simulink library "tqd"  (R2021b)
settings: Solver=VariableStepAuto  StartTime=0.0  StopTime=10.0  RelTol=1e-3
undefined symbols (not defined in the file or in its folder): ATQD_AccelLimitInRange_X_rpm, ATQD_AccelLimitInRange_Y_Nm, ATQD_AccelLimitOvrKi_X_Nm, ATQD_AccelLimitOvrKp_X_Nm, ATQD_BOSMapD_X_rpm, ATQD_BOSMapD_Y_pct, ATQD_BOSMapR_X_rpm, ATQD_BOSMapR_Y_pct, ATQD_HVBCurrSmooth_X_A, ATQD_LHMTqMapDLC_X_rpm, ATQD_LHMTqMapDLC_Y_pct, ATQD_LHMTqMapRLC_X_rpm, ATQD_LHMTqMapRLC_Y_pct, ATQD_NormalMapDLC_X_rpm, ATQD_NormalMapDLC_Y_pct, ATQD_NormalTqDecSR_X_rpm, ATQD_NormalTqDecSR_Y_Nm, ATQD_NormalTqIncSR_X_rpm, ATQD_NormalTqIncSR_Y_Nm, ATQD_OPDMapRLC_X_rpm, ATQD_OPDMapRLC_Y_pct, ATQD_RollRegTorReq_X_rpm, ATQD_RollRegTorReq_Y_enum, ATQD_VehSpdLimitInRange_X_rpm, ATQD_VehSpdLimitInRange_Y_Nm, ATQD_VehSpdLimitOvrKi_X_Nm, ATQD_VehSpdLimitOvrKp_X_Nm, EIGHT_INT, ENUM_BRAKEPEDAL_PRESSED, ENUM_BRAKEPEDAL_RELEASED, ENUM_COMBOKEY_DOWN, ENUM_COMBOKEY_M1, ENUM_COMBOKEY_M2, ENUM_COMBOKEY_NONE, ENUM_COMBOKEY_RKNEE, ENUM_COMBOKEY_STOPLV, ENUM_COMBOKEY_UP, ENUM_CP2VKNEEREQ_REQUEST, ENUM_CP2VNLVREQ_LEVEL1, ENUM_CP2VNLVREQ_LEVEL2, ENUM_CP2VNLVREQ_LOWER, ENUM_CP2VNLVREQ_STOPLV, ENUM_CP2VNLVREQ_UPPER, ENUM_CREEPIND_DISABLE, ENUM_CREEPIND_READY, ENUM_CREEPIND_RUNNING, ENUM_CREEPIND_WARNING, ENUM_DRIVELINERELEASE_RELEASE, ENUM_EBSTORQUERWQ_LIMIT, ENUM_EBSTORQUERWQ_TORQUE, ENUM_ECPVCUDRM_CONFORT, ENUM_ECPVCUDRM_ECO, ENUM_ECPVCUDRM_NORMAL, ENUM_ECPVCUDRM_NOTAVAILABLE, ENUM_EMTqModeDrvBrk_Accel, ENUM_EMTqModeDrvBrk_Brake, ENUM_EMTqModeDrvBrk_Coast, ENUM_ETC2ACTDRIVEDIR_BACKWARD, ENUM_ETC2ACTDRIVEDIR_FORWARD, ENUM_ETC2ACTDRIVEDIR_STILL ... (+341)
libraries: simulink x109, hcu_lib x67
(part 3 of 13)

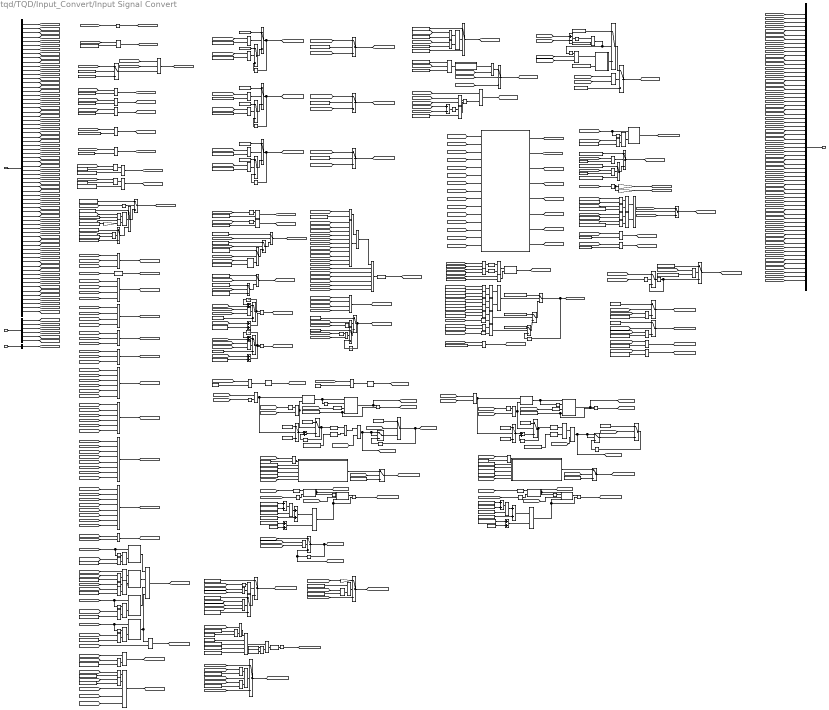
== system tqd/TQD/Input_Convert/Input Signal Convert ==
  note: VCU Vehicle Speed
  note: Motor Speed with Direction
  note: EBS Torque Control Determination
  note: Actual Driver Mode Determination
  note: Available Torque Calculation
  note: Target Shafter Speed Determination
  note: Gear Shifter Transfer Determination
  note: Gear Limitation with DMS Lost Communication
  note: DDM for DCQ
  note: Combo Key
  note: Engineering Mode Detection
  note: MCU Speed High Value Determination
  note: Actual Driving Direction Determination
  note: Power Limit/Gear Flash Indication Determination
  note: EBS Torque Request Determination
  note: IGN Active
  note: EV Drive Ready Judgment
  note: Gear Request Determination
  note: Door Open Judgment
  note: Brake Switch On
  note: Acceleration Pedal Depressed
  note: SCP Door Status
  note: Torque Source Determination
  BSCPIn_outputs : Inport
  BDCQ_Function_outputs : Inport  Port=2
  BDCQ_main_outputs : Inport  Port=3
  AND{,1..7,11..17} (15 alike) : Logic  AllPortsSameDT=off  OutDataTypeStr=boolean
  AND10 : Logic  Operator=OR  AllPortsSameDT=off  OutDataTypeStr=boolean
  AND18 : Logic  Inputs=3  AllPortsSameDT=off  OutDataTypeStr=boolean
  AND8 : Logic  Inputs=3  AllPortsSameDT=off  OutDataTypeStr=boolean
  AND9 : Logic  Operator=OR  AllPortsSameDT=off  OutDataTypeStr=boolean
  Abs{,1,5..6} (4 alike) : Abs
  Add{,1..3,7..14} (12 alike) : Sum
  Add5 : Sum  Inputs=+-
  Add6 : Sum  Inputs=+-
  "Big Mike Combo V2 " : Subsystem  TreatAsAtomicUnit=on
      settings: RTWSystemCode=Nonreusable function
  Bus Creator : BusCreator  Inputs=65
  Bus Selector : BusSelector  OutputSignals=task_time_s,VDHP_LowIdleAccPedal_flg,VINP_EBSBrakeSw_enum,VINP_TransReqGear_enum,VPMM_DrivelineRelease_enum,VPSA_Keystatus_enum,VINP_EM1ReqTorqLimDriv_pct,VINP_EM1ReqTorqLimBrk_pct,VPMM_SysPowerMode_enum,VDMM_DTCBMSRlyNoFB_flg,VDMM_DTCDCDCInverNoFB_flg,VDMM_DTCEACInverNoFB_flg,VDMM_DTCEACRlyNoFB_flg,VDMM_DTCEHPSInverNoFB_flg,VDMM_DTCEHPSRlyNoFB_flg,VDMM_DTCMCUHVRlyNoFB_flg,VDMM_DTCMCUIGBNoFB_flg,VDMM_DTCMCUCtrlMdNoFB_flg,VDMM_DTCACHVRlyNoFB_flg,VDMM_DTCMotorSpdNoFB_flg,VDMM_DTCMotorTrqNoFB_flg,VDMM_DTCDCDCRlyNoFB_flg,VDMM_DTCLostTC1_flg,VDMM_DTCDMSRCIncorrect_flg,VINP_MotorSpd_rpm,VINP_MotorSpdValid_flg,VINP_ECPVCUSpdLim_kph,VINP_ECPVCUSpdLimSw_flg,VINP_ParkBrakeSW_flg,VINP_BrakePedalPos_pct,VDHP_ActAPSPosn_pct,VDMM_DTCLostB2VST1_flg,VDMM_DTCLostB2VST2_flg,VDMM_DTCLostB2VCurrentLimit_flg,VDMM_DTCLostEMCEM1_flg,VDMM_DTCLostEBC1_flg,VDMM_DTCLostEBC2_flg,VDMM_DTCLostEBC5_flg,VDMM_ActLostEMCEM1_flg,VDMM_ActLostEBC1_flg,VDMM_ActLostEBC2_flg,VDMM_ActLostEBC5_flg,VDMM_ActLostMCUSta1_flg,VDMM_ActLostMCUSta2_flg,VDMM_ActLostMCUSta3_flg,VDMM_ActLostB2VST1_flg,VDMM_ActLostB2VST2_flg,VDMM_ActLostB2VCurrentLimit_flg,VDMM_DTCBCURCIncorrect_flg,VDMM_DTCPDURCIncorrect_flg,VINP_ECPVCUDRM_enum,VDMM_CAN1BUSOFF_flg,VINP_EM1OvrCtrlMDriv_enum,VINP_EM1OvrCtrlMBrk_enum,VDMM_EBSRCIncorrect_flg,VINP_FRHalbrakeReq_enum,VINP_MDHalbrakeReq_enum,VINP_TDHalbrakeReq_enum,VBCM_FDCBCMFDoorSta_flg,VBCM_FDCBCMMDoorSta_flg,VBCM_FDCBCMRDoorSta_flg,VACC_ASC2NLvReqFA_enum,VACC_ASC2NLvReqRA_enum,VACC_ASC2KneeReqRSide_flg,VACC_ASC2KneeReqFA_flg,VACC_ASC2KneeReqRA_flg,VBCM_FDCBCMFDCloseSVCmd_flg,VBCM_FDCBCMFDOpenSVCmd_flg,VINP_FASpeed_kph,VINP_CANMsgValidEBC2_flg
  Bus Selector1 : BusSelector  OutputSignals=VTQD_GearActualPosn_enum,VTQD_ParkingProtectWarning_flg,VTQD_TorqLimDoorOpn_flg,VTQD_VCUMCUCtrlMdTQD_enum,VTQD_TMTqCapMot_Nm,VTQD_TMTqCapGen_Nm
  Bus Selector2 : BusSelector  OutputSignals=VTQD_RrRampTq_Nm
  Constant{,2,71,73} (4 alike) : Constant  Value=ZERO_FLOAT
  Constant1 : Constant  Value=ENUM_GEARSHIFTPOSN_D
  Constant10 : Constant  Value=ENUM_BRAKEPEDAL_PRESSED
  Constant100 : Constant  Value=ENUM_MCUCTRLMODE_TORQUE
  Constant101 : Constant  Value=ENUM_GEARACTUALPOSN_R
  Constant102 : Constant  Value=KTQD_AbsoluteMotorSpdDir_flg
  Constant103 : Constant  Value=EPS
  Constant104 : Constant  Value=ENUM_GEARACTUALPOSN_N
  Constant105 : Constant  Value=ENUM_GEARACTUALPOSN_R
  Constant106 : Constant  Value=ENUM_GEARSHIFTPOSN_D
  Constant107 : Constant  Value=ENUM_GEARSHIFTPOSN_INVALID
  Constant108 : Constant  Value=ENUM_GEARSHIFTPOSN_N
  Constant109 : Constant  Value=ENUM_GEARSHIFTPOSN_R
  Constant11 : Constant  Value=ONE_PERCENT
  Constant110 : Constant  Value=KTQD_GearFlashSetTime_s
  Constant111 : Constant  Value=EPS
  Constant112 : Constant  Value=ENUM_GEARSHIFTPOSN_N
  Constant113 : Constant  Value=ENUM_GEARSHIFTPOSN_R
  Constant114 : Constant  Value=KTQD_VehSpdGearRatio_ratio
  Constant115 : Constant  Value=KTQD_ActDrvDirMotorSpdLimit_rpm  OutDataTypeStr=single
  Constant116 : Constant  Value=KTQD_GearFlashSetTime_s
  Constant117 : Constant  Value=EPS  OutDataTypeStr=single
  Constant118 : Constant  Value=KTQD_VehSpdTireFactor_Factor
  Constant119 : Constant  Value=KTQD_VehSpdTireDiameter_m
  Constant12 : Constant  Value=KTQD_MCUMaxRefTorq_Nm
  Constant120 : Constant  Value=KTQD_VehSpdADJFactor_Factor
  Constant{121,206,210,215,220} (5 alike) : Constant  Value=TRUE
  Constant122 : Constant  Value=SIXTY
  Constant123 : Constant  Value=THOUSAND
  Constant124 : Constant  Value=EPS  OutDataTypeStr=single
  Constant125 : Constant  Value=KTQD_TMSpd2FASpd_kph
  Constant126 : Constant  Value=KTQD_VCUVehSpdErr_kph
  Constant13 : Constant  Value=ENUM_GEARACTUALPOSN_D  OutDataTypeStr=Inherit: Inherit via back propagation
  Constant14 : Constant  Value=ENUM_GEARACTUALPOSN_P  OutDataTypeStr=Inherit: Inherit via back propagation
  Constant15 : Constant  Value=KTQD_EnLVChrgModekeyDet_s  OutDataTypeStr=single
  Constant16 : Constant  Value=ENUM_TARGETGEAR_DRIVE
  Constant17 : Constant  Value=ENUM_TARGETGEAR_NEUTRAL
  Constant176 : Constant  Value=uint8(6)
  Constant18 : Constant  Value=ENUM_TARGETGEAR_REVERSE
  Constant189 : Constant  Value=ENUM_VEHACTDRVDIR_ERROR
  Constant19 : Constant  Value=KTQD_EnLVChrgModeUION_s  VectorParams1D=off
  Constant198 : Constant  Value=KTQD_SpdLimSatHi_kph
  Constant20 : Constant  Value=KTQD_TDDoorSW_flg
  Constant200 : Constant  Value=KTQD_SpdLimSatLo_kph
  Constant202 : Constant  Value=KTQD_SpdLimDiv_rpm
  Constant{3,21,49..50,90,98,203,211,216,221} (10 alike) : Constant  Value=FALSE
  Constant204 : Constant  Value=KTQD_SpdLimDiv_rpm
  Constant205 : Constant  Value=KTQD_SpdLimIndFlash_cnt
  Constant207 : Constant  Value=KTQD_DoorStaSourceSW_flg
  Constant208 : Constant  Value=ENUM_HALBRAKEREQ_NOTACTIVE
  Constant209 : Constant  Value=ENUM_HALBRAKEREQ_ACTIVE
  Constant212 : Constant  Value=KTQD_DoorStaSourceSW_flg
  Constant213 : Constant  Value=ENUM_HALBRAKEREQ_NOTACTIVE
  Constant214 : Constant  Value=ENUM_HALBRAKEREQ_ACTIVE
  Constant217 : Constant  Value=KTQD_DoorStaSourceSW_flg
  Constant218 : Constant  Value=ENUM_HALBRAKEREQ_NOTACTIVE
  Constant219 : Constant  Value=ENUM_HALBRAKEREQ_ACTIVE
  Constant22 : Constant  Value=ENUM_KEYSTATUS_START
  Constant23 : Constant  Value=KTQD_DisLVChrgModeKeyDet_c  VectorParams1D=off
  Constant{24,44,52,55} (4 alike) : Constant  Value=ZERO_INT
  Constant242 : Constant  Value=ENUM_ECPVCUDRM_ECO
  Constant243 : Constant  Value=ENUM_ECPVCUDRM_CONFORT
  Constant244 : Constant  Value=KTQD_ECOComfortSpdLim_rpm
  Constant25 : Constant  Value=KTQD_EnLVChrgModeUIOFF_s  VectorParams1D=off
  Constant26 : Constant  Value=KTQD_EnLVChrgModeUIFlash_cnt  VectorParams1D=off
  Constant27 : Constant  Value=ENUM_DRIVELINERELEASE_RELEASE
  Constant28 : Constant  Value=KTQD_EnLVChrgModeUIWait_s  VectorParams1D=off
  Constant29 : Constant  Value=KTQD_EnLVChrgModeUION_s  VectorParams1D=off
  Constant30 : Constant  Value=KTQD_EnLVChrgModeUIOFF_s  VectorParams1D=off
  Constant31 : Constant  Value=KTQD_EnLVChrgModeUIFlash_cnt  VectorParams1D=off
  Constant32 : Constant  Value=KTQD_EnLVChrgModeUIWait_s  VectorParams1D=off
  Constant{33,47..48,54} (4 alike) : Constant  Value=ONE_INT
  Constant34 : Constant  Value=KTQD_EnLVChrgModeUITimes_cnt  VectorParams1D=off
  Constant35 : Constant  Value=FALSE  VectorParams1D=off
  Constant36 : Constant  Value=KTQD_DisLVChrgModeUION_s  VectorParams1D=off
  Constant37 : Constant  Value=KTQD_DisLVChrgModeUIOFF_s  VectorParams1D=off
  Constant38 : Constant  Value=KTQD_DisLVChrgModeUIFlash_cnt  VectorParams1D=off
  Constant39 : Constant  Value=KTQD_DisLVChrgModeUIWait_s  VectorParams1D=off
  Constant4 : Constant  Value=uint8(7)
  Constant40 : Constant  Value=KTQD_DisLVChrgModeUION_s  VectorParams1D=off
  Constant41 : Constant  Value=KTQD_DisLVChrgModeUIOFF_s  VectorParams1D=off
  Constant42 : Constant  Value=KTQD_DisLVChrgModeUIFlash_cnt  VectorParams1D=off
  Constant43 : Constant  Value=KTQD_DisLVChrgModeUIWait_s  VectorParams1D=off
  Constant45 : Constant  Value=KTQD_DisLVChrgModeUITimes_cnt  VectorParams1D=off
  Constant46 : Constant  Value=FALSE  VectorParams1D=off
  Constant5 : Constant  Value=KTQD_MCUMaxRefTorq_Nm
  Constant51 : Constant  Value=KTQD_EnLVChrgModeKeyDet_cnt
  Constant53 : Constant  Value=KTQD_DisLVChrgModeKeyDet_s  OutDataTypeStr=single
  Constant56 : Constant  Value=ENUM_GEARACTUALPOSN_R  OutDataTypeStr=Inherit: Inherit via back propagation
  Constant57 : Constant  Value=KTQD_VCUMCUDemHiPosVal_rpm
  Constant58 : Constant  Value=ENUM_TMROTATEDIRECTREQ_NONE  OutDataTypeStr=uint8
  Constant59 : Constant  Value=ENUM_TMROTATEDIRECTREQ_FWD  OutDataTypeStr=uint8
  Constant6 : Constant  Value=ONE_PERCENT
  Constant60 : Constant  Value=ENUM_TMROTATEDIRECTREQ_REV  OutDataTypeStr=uint8
  Constant61 : Constant  Value=KTQD_RotaDirRngUpTq_Nm
  Constant62 : Constant  Value=ENUM_GEARACTUALPOSN_R  OutDataTypeStr=Inherit: Inherit via back propagation
  Constant63 : Constant  Value=ENUM_GEARACTUALPOSN_D  OutDataTypeStr=Inherit: Inherit via back propagation
  Constant64 : Constant  Value=ENUM_TMROTATEDIRECTREQ_NONE  OutDataTypeStr=Inherit: Inherit via back propagation
  Constant65 : Constant  Value=ENUM_GEARACTUALPOSN_D
  Constant66 : Constant  Value=ENUM_TMROTATEDIRECTACT_REVERSE
  Constant67 : Constant  Value=ENUM_GEARACTUALPOSN_R
  Constant68 : Constant  Value=ENUM_PMMMODE_DRIVE
  Constant69 : Constant  Value=ENUM_TMROTATEDIRECTACT_FORWARD
  Constant{7,83..86} (5 alike) : Constant  Value=KTQD_ComLostTorqLimitRcv_kph
  Constant70 : Constant  Value=ONE_FLOAT
  Constant72 : Constant  Value=ENUM_TMROTATEDIRECTACT_FORWARD
  Constant74 : Constant  Value=ENUM_TMROTATEDIRECTACT_REVERSE
  Constant75 : Constant  Value=ENUM_TMROTATEDIRECTACT_NONE
  Constant76 : Constant  Value=ONE_FLOAT
  Constant77 : Constant  Value=ENUM_ECPVCUDRM_NOTAVAILABLE
  Constant78 : Constant  Value=ENUM_ECPVCUDRM_NORMAL
  Constant79 : Constant  Value=ENUM_TQSOURCE_INTERNAL
  Constant8 : Constant  Value=ENUM_GEARACTUALPOSN_N  OutDataTypeStr=Inherit: Inherit via back propagation
  Constant80 : Constant  Value=KTQD_DMSLostTorqLimit_kph
  Constant81 : Constant  Value=ENUM_TQSOURCE_ESC
  Constant82 : Constant  Value=ENUM_TQSOURCE_LIMIT
  Constant87 : Constant  Value=KTQD_ActDrvDirMotorSpdLimit_rpm  OutDataTypeStr=single
  Constant88 : Constant  Value=KTQD_ActDrvDirMotorSpdLimit_rpm  OutDataTypeStr=single
  Constant89 : Constant  Value=KTQD_CAN1BusOffSpdRcv_kph
  Constant9 : Constant  Value=KTQD_RotaDirRngLowTq_Nm
  Constant91 : Constant  Value=ENUM_VEHACTDRVDIR_STILL
  Constant92 : Constant  Value=ENUM_EBSTORQUERWQ_TORQUE
  Constant93 : Constant  Value=ENUM_VEHACTDRVDIR_FORWARD
  Constant94 : Constant  Value=ENUM_EBSTORQUERWQ_LIMIT
  Constant95 : Constant  Value=ENUM_VEHACTDRVDIR_BACKWARD
  Constant96 : Constant  Value=ENUM_EBSTORQUERWQ_TORQUE
  Constant97 : Constant  Value=ENUM_EBSTORQUERWQ_LIMIT
  Constant99 : Constant  Value=ENUM_GEARACTUALPOSN_N
  Data Type Conversion : DataTypeConversion  OutDataTypeStr=boolean
  Data Type Conversion1 : DataTypeConversion  OutDataTypeStr=single
  Data Type Conversion2 : DataTypeConversion  OutDataTypeStr=single
  Data Type Conversion3 : DataTypeConversion  OutDataTypeStr=single
  Data Type Conversion{4,6..8} (4 alike) : DataTypeConversion  OutDataTypeStr=uint16
  Data Type Conversion5 : DataTypeConversion  OutDataTypeStr=boolean
  Delay : Delay  DelayLength=1  InitialConditionSource=Input port
      settings: AttributesFormatString=%<InitialConditionSource>  InputPortMap=u0,p4
  Delay{1..3,8..9,11..15} (10 alike) : Delay  DelayLength=1  InitialCondition=boolean(0)
      settings: AttributesFormatString=%<InitialCondition>
  Delay{4..7,10} (5 alike) : Delay  DelayLength=1  InitialCondition=uint8(0)
      settings: AttributesFormatString=%<InitialCondition>
  Detect Change2 : simulink/Logic and Bit Operations/Detect Change  vinit=boolean(0)  OutDataTypeStr=uint8
  Detect Change3 : simulink/Logic and Bit Operations/Detect Change  vinit=boolean(0)  OutDataTypeStr=uint8
  Detect Decrease : simulink/Logic and Bit Operations/Detect Decrease  vinit=boolean(0)  OutDataTypeStr=boolean
  Detect Increase : simulink/Logic and Bit Operations/Detect Increase  vinit=boolean(0)  OutDataTypeStr=boolean
  Detect Rise Positive1 : simulink/Logic and Bit Operations/Detect Rise Positive  vinit=boolean(0)  OutDataTypeStr=boolean
  Detect Rise Positive2 : simulink/Logic and Bit Operations/Detect Rise Positive  vinit=boolean(0)  OutDataTypeStr=boolean
  Divide : Product  Inputs=**
  Divide1 : Product  Inputs=**
  Divide2 : Product  Inputs=*/
  Divide3 : Product  Inputs=*/
  Engineering Mode Disable Flasher : Subsystem
      settings: RTWSystemCode=Nonreusable function
  Engineering Mode Enable Flasher : Subsystem
      settings: RTWSystemCode=Nonreusable function
  Equal{,1..7,9..10,12,14..18,21,31,34..39,48..49} (26 alike) : RelationalOperator  Operator===  OutDataTypeStr=boolean  RndMeth=Simplest
  Equal11 : RelationalOperator  Operator=>  OutDataTypeStr=boolean  RndMeth=Simplest
  Equal13 : RelationalOperator  Operator=<  OutDataTypeStr=boolean  RndMeth=Simplest
  Equal8 : RelationalOperator  Operator=~=  OutDataTypeStr=boolean  RndMeth=Simplest
  Flasher : Subsystem
      settings: RTWSystemCode=Nonreusable function
  Gain : Gain  Gain=MINUS_ONE
  Gain1 : Gain  Gain=ONE_FLOAT
  Gain2 : Gain  Gain=MINUSONE_FLOAT
  Gain3 : Gain  Gain=MINUS_ONE
  LiuZgSwitch{1..2,4,6..8} (6 alike) : Switch  Criteria=u2 ~= 0  Threshold=0.5
      settings: AttributesFormatString=<%<Criteria>>
  Logical Operator{,1,3..5,7..11} (10 alike) : Logic  AllPortsSameDT=off  OutDataTypeStr=boolean
  Logical Operator2 : Logic  Operator=OR  AllPortsSameDT=off  OutDataTypeStr=boolean
  Logical Operator6 : Logic  Operator=OR  AllPortsSameDT=off  OutDataTypeStr=boolean
  Max{,1..3} (4 alike) : MinMax  Function=max  Inputs=2
  Min : MinMax  Inputs=2
  NOT{,1..18} (19 alike) : Logic  Operator=NOT  AllPortsSameDT=off  OutDataTypeStr=boolean
  OR{,2,5..6,18} (5 alike) : Logic  Operator=OR  Inputs=3  AllPortsSameDT=off  OutDataTypeStr=boolean
  OR{1,14..17,21} (6 alike) : Logic  Operator=OR  AllPortsSameDT=off  OutDataTypeStr=boolean
  OR10 : Logic  Operator=OR  Inputs=8  AllPortsSameDT=off  OutDataTypeStr=boolean
  OR{3..4,11,22} (4 alike) : Logic  Operator=OR  Inputs=4  AllPortsSameDT=off  OutDataTypeStr=boolean
  OR12 : Logic  Operator=OR  Inputs=7  AllPortsSameDT=off  OutDataTypeStr=boolean
  OR13 : Logic  Operator=OR  Inputs=11  AllPortsSameDT=off  OutDataTypeStr=boolean
  OR20 : Logic  AllPortsSameDT=off  OutDataTypeStr=boolean
  OR23 : Logic  Operator=OR  Inputs=5  AllPortsSameDT=off  OutDataTypeStr=boolean
  OR7 : Logic  Operator=OR  Inputs=6  AllPortsSameDT=off  OutDataTypeStr=boolean
  OR8 : Logic  Operator=OR  Inputs=6  AllPortsSameDT=off  OutDataTypeStr=boolean
  OR9 : Logic  Operator=OR  Inputs=8  AllPortsSameDT=off  OutDataTypeStr=boolean
  Product{,1..7} (8 alike) : Product
  Product8 : Product  Inputs=5
  RegenLV_inc2 : Constant  Value=KTQD_DRTransferRestTq_Nm
  Relational Operator{,3,10,12,14..15,34} (7 alike) : RelationalOperator  OutDataTypeStr=boolean  RndMeth=Simplest
  Relational Operator{1,4,8,29..33,38} (9 alike) : RelationalOperator  Operator=<=  OutDataTypeStr=boolean  RndMeth=Simplest
  Relational Operator11 : RelationalOperator  Operator===  OutDataTypeStr=boolean  RndMeth=Simplest
  Relational Operator13 : RelationalOperator  Operator===  OutDataTypeStr=boolean  RndMeth=Simplest
  Relational Operator{2,16..18,21..22,24..28,35} (12 alike) : RelationalOperator  Operator===  OutDataTypeStr=boolean  RndMeth=Nearest
  Relational Operator19 : RelationalOperator  Operator=<=  OutDataTypeStr=boolean  RndMeth=Nearest
  Relational Operator20 : RelationalOperator  OutDataTypeStr=boolean  RndMeth=Nearest
  Relational Operator23 : RelationalOperator  Operator=<=  OutDataTypeStr=boolean  RndMeth=Nearest
  Relational Operator36 : RelationalOperator  Operator=~=  OutDataTypeStr=boolean  RndMeth=Nearest
  Relational Operator37 : RelationalOperator  Operator=>  OutDataTypeStr=boolean  RndMeth=Simplest
  Relational Operator5 : RelationalOperator  OutDataTypeStr=boolean  RndMeth=Nearest
  Relational Operator6 : RelationalOperator  Operator=>  OutDataTypeStr=boolean  RndMeth=Simplest
  Relational Operator7 : RelationalOperator  Operator=<  OutDataTypeStr=boolean  RndMeth=Nearest
  Relational Operator9 : RelationalOperator  Operator=>  OutDataTypeStr=boolean  RndMeth=Nearest
  SR_Latch{,1..3,5..10} (10 alike) : hcu_lib/Basic_Blocks/SR_Latch
      SR_Latch5 settings: SourceProductName=HCU Relative Block Library
      SR_Latch6 settings: SourceProductName=HCU Relative Block Library
  Saturation Dynamic : simulink/Discontinuities/Saturation Dynamic  OutMin=[]  OutMax=[]  OutDataTypeStr=Inherit: Same as second input  OutDataType=fixdt(1, 16)  OutScaling=2^-10  DoSatur=off
  Switch{,2..9,11..28,67..69,87..98,107} (43 alike) : Switch  Criteria=u2 ~= 0
      settings: AttributesFormatString=%<Criteria>
  Switch1 : Switch  Criteria=u2 ~= 0  Threshold=0.5
      settings: AttributesFormatString=%<Criteria>
  Switch10 : Switch  Criteria=u2 > Threshold
  Timer{1..4} (4 alike) : hcu_lib/Basic_Blocks/Timer
  Unit Delay : UnitDelay  InitialCondition=single(0)  SampleTime=-1  HasFrameUpgradeWarning=on
      settings: AttributesFormatString=%<InitialCondition>
  Unit Delay1 : UnitDelay  InitialCondition=uint8(0)  SampleTime=-1
      settings: AttributesFormatString=%<InitialCondition>
  Unit Delay3 : UnitDelay  InitialCondition=single(0)  SampleTime=-1  HasFrameUpgradeWarning=on
      settings: AttributesFormatString=%<InitialCondition>
  Unit Delay4 : UnitDelay  InitialCondition=boolean(0)  SampleTime=-1  HasFrameUpgradeWarning=on
      settings: AttributesFormatString=%<InitialCondition>
  "kph to rpm " : Subsystem
      settings: RTWSystemCode=Nonreusable function
  BSignalConvert_outputs : Outport
  wires:
  BSCPIn_outputs/1 -> Bus Selector/1
  NOT/1 -> [VTQD_AccelPedalDepressed_flg]  "VTQD_AccelPedalDepressed_flg"
  [VDHP_LowIdleAccPedal_flg] -> NOT/1
  [VINP_EBSBrakeSw_enum] -> Equal1/1
  Equal1/1 -> [VTQD_BrkSWOn_flg]  "VTQD_BrkSWOn_flg"
  Constant10/1 -> Equal1/2
  Constant20/1 -> Switch2/2
  [VTQD_ActTDDoorOPSta_flg] -> Switch2/1
  Switch2/1 -> OR/3
  [VTQD_ActFRDoorOPSta_flg] -> OR/2
  OR/1 -> [VTQD_DoorOpen_flg]  "VTQD_DoorOpen_flg"
  [VTQD_ActMDDoorOPSta_flg] -> OR/1
  Constant21/1 -> Switch2/3
  Constant16/1 -> Equal4/2
  Equal6/1 -> [VTQD_ReversePositionOn_flg]  "VTQD_ReversePositionOn_flg"
  Constant17/1 -> Equal5/2
  [VINP_TransReqGear_enum] -> Equal6/1
  [VINP_TransReqGear_enum] -> Equal4/1
  Equal4/1 -> [VTQD_DrivePositionOn_flg]  "VTQD_DrivePositionOn_flg"
  Equal5/1 -> [VTQD_NeutralPositionOn_flg]  "VTQD_NeutralPositionOn_flg"
  Constant18/1 -> Equal6/2
  [VINP_TransReqGear_enum] -> Equal5/1
  Equal12/1 -> [VTQD_EVDriveReady_flg]  "VTQD_EVDriveReady_flg"
  [VPMM_DrivelineRelease_enum] -> Equal12/1
  Constant27/1 -> Equal12/2
  Equal9/1 -> [VTQD_IGNActive_flg]  "VTQD_IGNActive_flg"
  Constant22/1 -> Equal9/2
  [VPSA_Keystatus_enum] -> Equal9/1
  Constant12/1 -> Product/2
  [VINP_EM1ReqTorqLimBrk_pct] -> Product3/1
  [VINP_EM1ReqTorqLimDriv_pct] -> Product2/1
  Product1/1 -> [VTQD_EM1ReqTorqLimBrk_Nm]  "VTQD_EM1ReqTorqLimBrk_Nm"
  Constant5/1 -> Product1/2
  Product3/1 -> Product1/1
  Product/1 -> [VTQD_EM1ReqTorqLimDriv_Nm]  "VTQD_EM1ReqTorqLimDriv_Nm"
  Constant6/1 -> Product2/2
  Product2/1 -> Product/1
  Constant11/1 -> Product3/2
  Switch97/1 -> Switch98/3
  Constant212/1 -> Switch93/2
  Equal39/1 -> Switch98/2
  Delay1/1 -> Switch91/3
  [VTQD_MDHalbrakeReq_flg] -> Switch93/1
  [VTQD_FRHalbrakeReq_flg] -> Switch90/1
  Equal34/1 -> Switch91/2
  Switch98/1 -> [VTQD_TDHalbrakeReq_flg], Delay3/1  "VTQD_TDHalbrakeReq_flg"
  Delay2/1 -> Switch94/3
  Switch92/1 -> [VTQD_FRHalbrakeReq_flg], Delay1/1  "VTQD_FRHalbrakeReq_flg"
  Constant218/1 -> Equal39/2
  Constant221/1 -> Switch98/1
  Constant216/1 -> Switch95/1
  Constant219/1 -> Equal38/2
  Switch94/1 -> Switch95/3
  Constant214/1 -> Equal36/2
  Equal38/1 -> Switch97/2
  Equal36/1 -> Switch94/2
  Constant209/1 -> Equal34/2
  Switch96/1 -> [VTQD_ActTDDoorOPSta_flg]  "VTQD_ActTDDoorOPSta_flg"
  Constant220/1 -> Switch97/1
  Constant217/1 -> Switch96/2
  [VTQD_TDHalbrakeReq_flg] -> Switch96/1
  Switch95/1 -> Delay2/1, [VTQD_MDHalbrakeReq_flg]  "VTQD_MDHalbrakeReq_flg"
  Equal37/1 -> Switch95/2
  Constant215/1 -> Switch94/1
  Switch93/1 -> [VTQD_ActMDDoorOPSta_flg]  "VTQD_ActMDDoorOPSta_flg"
  Constant211/1 -> Switch92/1
  Constant210/1 -> Switch91/1
  Equal35/1 -> Switch92/2
  Constant208/1 -> Equal35/2
  Switch91/1 -> Switch92/3
  Constant213/1 -> Equal37/2
  Constant207/1 -> Switch90/2
  Delay3/1 -> Switch97/3
  Switch90/1 -> [VTQD_ActFRDoorOPSta_flg]  "VTQD_ActFRDoorOPSta_flg"
  Bus Selector/2 -> [VDHP_LowIdleAccPedal_flg]  "<VDHP_LowIdleAccPedal_flg>"
  [VINP_FRHalbrakeReq_enum] -> Equal35/1
  [VINP_FRHalbrakeReq_enum] -> Equal34/1
  [VBCM_FDCBCMFDoorSta_flg] -> Switch90/3
  [VINP_MDHalbrakeReq_enum] -> Equal37/1
  [VINP_MDHalbrakeReq_enum] -> Equal36/1
  [VBCM_FDCBCMMDoorSta_flg] -> Switch93/3
  [VINP_TDHalbrakeReq_enum] -> Equal39/1
  [VINP_TDHalbrakeReq_enum] -> Equal38/1
  [VBCM_FDCBCMRDoorSta_flg] -> Switch96/3
  Equal7/1 -> [VTQD_GearInR_flg]  "VTQD_GearInR_flg"
  Equal3/1 -> [VTQD_GearInN_flg]  "VTQD_GearInN_flg"
  Constant106/1 -> Switch12/1
  [VTQD_DrivePositionOn_flg] -> Switch12/2
  [VTQD_GearInN_flg] -> Switch16/2
  Switch12/1 -> Switch13/3
  Switch13/1 -> Switch14/3
  Switch17/1 -> [VTQD_RealGear_enum]  "VTQD_RealGear_enum"
  Constant1/1 -> Switch16/3
  Constant107/1 -> Delay/2
  Delay/1 -> Switch12/3
  [VTQD_ReversePositionOn_flg] -> Switch14/2
  Switch16/1 -> Switch17/3
  Constant108/1 -> Switch13/1
  Constant109/1 -> Switch14/1
  Switch14/1 -> [VTQD_ReqGear_enum]  "VTQD_ReqGear_enum"
  [VTQD_NeutralPositionOn_flg] -> Switch13/2
  [VTQD_GearInR_flg] -> Switch17/2
  Constant113/1 -> Switch17/1
  Constant112/1 -> Switch16/1
  Bus Selector/3 -> [VINP_EBSBrakeSw_enum]  "<VINP_EBSBrakeSw_enum>"
  Bus Selector/4 -> [VINP_TransReqGear_enum]  "<VINP_TransReqGear_enum>"
  Bus Selector/5 -> [VPMM_DrivelineRelease_enum]  "<VPMM_DrivelineRelease_enum>"
  Bus Selector/6 -> [VPSA_Keystatus_enum]  "<VPSA_Keystatus_enum>"
  Bus Selector/7 -> [VINP_EM1ReqTorqLimDriv_pct]  "<VINP_EM1ReqTorqLimDriv_pct>"
  Bus Selector/8 -> [VINP_EM1ReqTorqLimBrk_pct]  "<VINP_EM1ReqTorqLimBrk_pct>"
  [VTQD_ReqGear_enum] -> Delay/1
  Equal8/1 -> Switch18/2
  Constant/1 -> Switch18/3
  Unit Delay/1 -> Add/1
  Constant116/1 -> Add1/2
  Add1/1 -> Relational Operator/2
  Constant110/1 -> Add3/2
  Relational Operator3/1 -> [OnOffDebounce]  "OnOffDebounce"
  Switch25/1 -> Unit Delay3/1, Relational Operator3/1
  Add3/1 -> Relational Operator3/2
  [VTQD_ReqGear_enum] -> Equal8/1
  Add/1 -> Switch18/1
  Equal2/1 -> Switch25/2
  Relational Operator/1 -> [OffOnDebounce]  "OffOnDebounce"
  Switch18/1 -> Relational Operator/1, Unit Delay/1
  [task_time_s] -> Add2/2
  [VTQD_ReqGear_enum] -> Equal2/1
  Unit Delay3/1 -> Add2/1
  Add2/1 -> Switch25/1
  [VTQD_RealGear_enum] -> Equal8/2
  [VTQD_RealGear_enum] -> Equal2/2
  Bus Selector/1 -> [task_time_s]  "<task_time_s>"
  [task_time_s] -> Add/2
  [task_time_s] -> Add1/1
  [task_time_s] -> Add3/1
  Constant2/1 -> Switch25/3
  Constant68/1 -> Equal21/2
  Equal21/1 -> AND3/1
  AND3/1 -> OR12/1
  [VDMM_DTCMotorSpdNoFB_flg] -> OR12/2
  Logical Operator1/1 -> Switch27/2
  [VPMM_SysPowerMode_enum] -> Equal21/1
  Data Type Conversion5/1 -> [VTQD_VCU4PweLmtInd_flg]  "VTQD_VCU4PweLmtInd_flg"
  OR13/1 -> AND3/2
  [VDMM_DTCMotorTrqNoFB_flg] -> OR12/3
  OR12/1 -> Data Type Conversion5/1
  Unit Delay4/1 -> Switch27/3
  OR11/1 -> [VTQD_GearFlashIndDis_flg]  "VTQD_GearFlashIndDis_flg"
  Logical Operator/1 -> Switch26/2
  Switch27/1 -> Switch26/3
  Switch26/1 -> [VTQD_GearFlashInd_flg], Unit Delay4/1  "VTQD_GearFlashInd_flg"
  Bus Selector/9 -> [VPMM_SysPowerMode_enum]  "<VPMM_SysPowerMode_enum>"
  Bus Selector/10 -> [VDMM_DTCBMSRlyNoFB_flg]  "<VDMM_DTCBMSRlyNoFB_flg>"
  Bus Selector/11 -> [VDMM_DTCDCDCInverNoFB_flg]  "<VDMM_DTCDCDCInverNoFB_flg>"
  Bus Selector/12 -> [VDMM_DTCEACInverNoFB_flg]  "<VDMM_DTCEACInverNoFB_flg>"
  Bus Selector/13 -> [VDMM_DTCEACRlyNoFB_flg]  "<VDMM_DTCEACRlyNoFB_flg>"
  Bus Selector/14 -> [VDMM_DTCEHPSInverNoFB_flg]  "<VDMM_DTCEHPSInverNoFB_flg>"
  Bus Selector/15 -> [VDMM_DTCEHPSRlyNoFB_flg]  "<VDMM_DTCEHPSRlyNoFB_flg>"
  Bus Selector/16 -> [VDMM_DTCMCUHVRlyNoFB_flg]  "<VDMM_DTCMCUHVRlyNoFB_flg>"
  Bus Selector/17 -> [VDMM_DTCMCUIGBNoFB_flg]  "<VDMM_DTCMCUIGBNoFB_flg>"
  Bus Selector/18 -> [VDMM_DTCMCUCtrlMdNoFB_flg]  "<VDMM_DTCMCUCtrlMdNoFB_flg>"
  Bus Selector/19 -> [VDMM_DTCACHVRlyNoFB_flg]  "<VDMM_DTCACHVRlyNoFB_flg>"
  Bus Selector/20 -> [VDMM_DTCMotorSpdNoFB_flg]  "<VDMM_DTCMotorSpdNoFB_flg>"
  Bus Selector/21 -> [VDMM_DTCMotorTrqNoFB_flg]  "<VDMM_DTCMotorTrqNoFB_flg>"
  [VDMM_DTCBMSRlyNoFB_flg] -> OR13/1
  [VDMM_DTCDCDCInverNoFB_flg] -> OR13/2
  [VDMM_DTCEACInverNoFB_flg] -> OR13/3
  [VDMM_DTCEACRlyNoFB_flg] -> OR13/4
  [VDMM_DTCEHPSInverNoFB_flg] -> OR13/5
  [VDMM_DTCEHPSRlyNoFB_flg] -> OR13/6
  [VDMM_DTCMCUHVRlyNoFB_flg] -> OR13/7
  [VDMM_DTCMCUIGBNoFB_flg] -> OR13/8
  [VDMM_DTCMCUCtrlMdNoFB_flg] -> OR13/9
  [VDMM_DTCACHVRlyNoFB_flg] -> OR13/10
  Bus Selector/22 -> [VDMM_DTCDCDCRlyNoFB_flg]  "<VDMM_DTCDCDCRlyNoFB_flg>"
  [VDMM_DTCDCDCRlyNoFB_flg] -> OR13/11
  [VDMM_CAN1BUSOFF_flg] -> OR12/4
  [VTQD_SpdLimInd_flg] -> OR12/5
  [VTQD_ParkingProtectWarning_flg] -> OR12/6
  [VTQD_TorqLimDoorOpn_flg] -> OR12/7
  Bus Selector/23 -> [VDMM_DTCLostTC1_flg]  "<VDMM_DTCLostTC1_flg>"
  Bus Selector/24 -> [VDMM_DTCDMSRCIncorrect_flg]  "<VDMM_DTCDMSRCIncorrect_flg>"
  [VDMM_DTCLostTC1_flg] -> OR11/1
  [VDMM_DTCDMSRCIncorrect_flg] -> OR11/2
  [VTQD_TorqLimDoorOpn_flg] -> OR11/3
  [VTQD_GearFlashInd_flg] -> OR11/4
  [OffOnDebounce] -> Logical Operator/1
  Constant121/1 -> Switch26/1
  Constant3/1 -> Switch27/1
  NOT1/1 -> Logical Operator/2
  [OnOffDebounce] -> NOT1/1
  [OnOffDebounce] -> Logical Operator1/2
  [OffOnDebounce] -> NOT2/1
  NOT2/1 -> Logical Operator1/1
  [VINP_MotorSpdValid_flg] -> NOT4/1
  [VINP_MotorSpd_rpm] -> Relational Operator9/1
  Gain/1 -> Relational Operator9/2
  Relational Operator9/1 -> Logical Operator8/2
  Constant189/1 -> Switch69/1
  Relational Operator5/1 -> Switch67/2
  Logical Operator8/1 -> Switch68/2
  Relational Operator7/1 -> Logical Operator8/1
  [VINP_MotorSpd_rpm] -> Relational Operator5/1
  Constant91/1 -> Switch68/1
  Switch68/1 -> Switch69/3
  Constant87/1 -> Relational Operator5/2
  Switch69/1 -> [VTQD_EVCU1VehActDrvDir_enum]  "VTQD_EVCU1VehActDrvDir_enum"
  Constant88/1 -> Gain/1
  [VINP_MotorSpd_rpm] -> Relational Operator7/1
  NOT4/1 -> Switch69/2
  Constant95/1 -> Switch67/3
  Constant93/1 -> Switch67/1
  Switch67/1 -> Switch68/3
  Constant115/1 -> Relational Operator7/2
  Bus Selector/25 -> [VINP_MotorSpd_rpm]  "<VINP_MotorSpd_rpm>"
  Bus Selector/26 -> [VINP_MotorSpdValid_flg]  "<VINP_MotorSpdValid_flg>"
  [VTQD_SpecSpdLim_rpm] -> Switch87/3
  "kph to rpm "/1(MotorSpd_rpm) -> Min/1  "VTQD_ECPCalSpdLimTG_rpm"
  Min/1 -> Switch87/1
  Constant200/1 -> Saturation Dynamic/3
  [VTQD_SpecSpdLim_rpm] -> Min/2
  Saturation Dynamic/1 -> "kph to rpm "/1(SetSpeed_kph)
  [VINP_ECPVCUSpdLimSw_flg] -> Switch87/2
  Constant198/1 -> Saturation Dynamic/1
  Switch87/1 -> [VTQD_VCUMCUDemHiPosVal_rpm]  "VTQD_VCUMCUDemHiPosVal_rpm"
  [VINP_ECPVCUSpdLim_kph] -> Saturation Dynamic/2
  Bus Selector/27 -> [VINP_ECPVCUSpdLim_kph]  "<VINP_ECPVCUSpdLim_kph>"
  Bus Selector/28 -> [VINP_ECPVCUSpdLimSw_flg]  "<VINP_ECPVCUSpdLimSw_flg>"
  Switch107/1 -> [VTQD_SpecSpdLim_rpm]  "VTQD_SpecSpdLim_rpm"
  Equal49/1 -> OR17/1
  Constant244/1 -> Switch107/1
  Constant242/1 -> Equal48/2
  Constant57/1 -> Switch107/3
  Equal48/1 -> OR17/2
  OR17/1 -> Switch107/2
  Constant243/1 -> Equal49/2
  [VTQD_ActDriveMode_enum] -> Equal49/1
  [VTQD_ActDriveMode_enum] -> Equal48/1
  Constant202/1 -> Relational Operator4/2
  AND6/1 -> [VTQD_SpdLimSta_flg]  "VTQD_SpdLimSta_flg"
  Abs5/1 -> Relational Operator4/1
  Relational Operator4/1 -> OR16/2
  [VTQD_VCUMCUDemHiPosVal_rpm] -> Add5/2
  Add5/1 -> Abs5/1
  [VTQD_VCUMCUDemHiPosVal_rpm] -> Relational Operator6/2
  Relational Operator6/1 -> OR16/1
  OR16/1 -> AND6/2  "VSCP_SpdInRange_flg"
  [VINP_ECPVCUSpdLimSw_flg] -> AND6/1
  [VINP_MotorSpd_rpm] -> Add5/1
  [VINP_MotorSpd_rpm] -> Relational Operator6/1
  AND8/1 -> Flasher/1(triger)
  [VTQD_SpdLimSta_flg] -> AND7/2
  Relational Operator8/1 -> NOT3/1, Switch89/2
  Flasher/1(Result) -> Switch89/3
  Switch88/1 -> [VTQD_SpdLimInd_flg]  "VTQD_SpdLimInd_flg"
  Switch89/1 -> Switch88/1
  Constant205/1 -> Flasher/2(FlashTime)
  Constant203/1 -> Switch88/3
  [VTQD_VCUMCUDemHiPosVal_rpm] -> Add6/2
  Constant204/1 -> Relational Operator8/2
  Abs6/1 -> Relational Operator8/1
  Add6/1 -> Abs6/1
  AND7/1 -> Switch88/2
  NOT3/1 -> AND8/1
  Constant206/1 -> Switch89/1
  [VTQD_SpdLimSta_flg] -> AND8/3
  [VINP_MotorSpd_rpm] -> Add6/1
  [VINP_ECPVCUSpdLimSw_flg] -> AND8/2
  [VINP_ECPVCUSpdLimSw_flg] -> AND7/1
  Constant32/1 -> Add10/2
  [VTQD_EngModeOffRiseDet_flg] -> AND10/2
  Delay8/1 -> AND10/1
  Add10/1 -> Product5/1  "VTQD_EnFlashCycleTime_s"
  [VTQD_InitLVchrgSvrMode_flg] -> Detect Decrease/1
  Constant36/1 -> Engineering Mode Disable Flasher/2(ON_s)
  NOT9/1 -> Timer3/2
  Constant37/1 -> Engineering Mode Disable Flasher/3(OFF_s)
  Constant38/1 -> Engineering Mode Disable Flasher/4(Cycle_cnt)
  Switch9/1 -> Delay10/1, Data Type Conversion4/1
  Detect Decrease/1 -> SR_Latch10/1
  Switch15/1 -> [VTQD_InitLVchrgSvrMode_flg], Delay9/1  "VTQD_InitLVchrgSvrMode_flg"
  Relational Operator12/1 -> [VTQD_EngModeDisDetEnd_flg]  "VTQD_EngModeDisDetEnd_flg"
  [task_time_s] -> Data Type Conversion3/1
  Constant53/1 -> Relational Operator12/2, Timer2/4
  [VTQD_EngModeDisDetEnd_flg] -> AND5/2
  [VTQD_EngModeDisDetEnd_flg] -> Delay11/1
  Constant55/1 -> Switch8/3
  NOT8/1 -> Timer2/2
  Switch8/1 -> Add8/1
  Delay9/1 -> Switch7/3
  NOT7/1 -> Timer1/2
  [VTQD_EngModeEnDetEnd_flg] -> Delay8/1
  Switch5/1 -> Delay7/1, Data Type Conversion7/1
  [VTQD_EngModeEnDetEnd_flg] -> AND2/2
  Add7/1 -> Switch5/3
  Data Type Conversion2/1 -> Timer1/3
  [task_time_s] -> Data Type Conversion2/1
  AND2/1 -> Switch7/2, Switch7/1, [VTQD_EngModeOnDelay_flg]  "VTQD_EngModeOnDelay_flg"
  Add8/1 -> Switch9/3
  AND5/1 -> Switch11/1, Switch11/2, [VTQD_EngModeOffDelay_flg]  "VTQD_EngModeOffDelay_flg"
  Add9/1 -> Product4/1
  AND10/1 -> SR_Latch1/2, Switch5/2
  [VTQD_EngModeOnRiseDet_flg] -> AND9/2
  SR_Latch1/1 -> NOT7/1, Timer1/1
  Constant24/1 -> Switch9/1
  AND9/1 -> SR_Latch2/2, Switch9/2
  Detect Increase/1 -> SR_Latch3/1
  [VTQD_InitLVchrgSvrMode_flg] -> Detect Increase/1
  Constant54/1 -> Switch8/1
  Relational Operator13/1 -> AND5/1
  Data Type Conversion3/1 -> Timer2/3
  Timer1/1 -> [VTQD_EngModeEnDetTime_s], Relational Operator10/1  "VTQD_EngModeEnDetTime_s"
  Add11/1 -> Product6/1
  [VTQD_EngModeEnFlashFinished_flg] -> OR1/2
  Delay7/1 -> Add7/2
  [VTQD_LVchrgSvrModeDelay_flg] -> NOT11/1
  Constant30/1 -> Add9/2
  Detect Rise Positive2/1 -> [VTQD_EngModeOnRiseDet_flg]  "VTQD_EngModeOnRiseDet_flg"
  Constant39/1 -> Engineering Mode Disable Flasher/5(Wait_s)
  Delay14/1 -> Switch21/3, [VTQD_LVchrgSvrModeDelay_flg]  "VTQD_LVchrgSvrModeDelay_flg"
  Switch20/1 -> [VTQD_AmberFlashOff_flg]  "VTQD_AmberFlashOff_flg"
  Relational Operator15/1 -> [VTQD_EngModeDisFlashFinished_flg]  "VTQD_EngModeDisFlashFinished_flg"
  Constant33/1 -> Switch4/1
  Constant28/1 -> Engineering Mode Enable Flasher/5(Wait_s)
  Relational Operator11/1 -> AND2/1
  Delay10/1 -> Add8/2
  OR1/1 -> Switch21/2
  Constant29/1 -> Add9/1
  Constant40/1 -> Add11/1
  Constant31/1 -> Product4/2
  Constant42/1 -> Product6/2
  Product7/1 -> Timer4/4, Relational Operator15/2
  [task_time_s] -> Timer4/3
  NOT10/1 -> Timer4/2
  Constant35/1 -> Switch19/3
  [VTQD_FlasherEn_flg] -> Switch19/2
  [VTQD_FlasherEn_flg] -> Engineering Mode Enable Flasher/6(VSCP_FlasherEn_flg)
  NOT11/1 -> AND11/2
  Engineering Mode Disable Flasher/1(SigOut) -> Switch20/1
  [VTQD_FlasherDis_flg] -> Engineering Mode Disable Flasher/6(VSCP_FlasherEn_flg)
  Constant41/1 -> Add11/2
  Switch10/1 -> Delay13/1
  SR_Latch3/1 -> Timer3/1, NOT9/1, [VTQD_FlasherEn_flg]  "VTQD_FlasherEn_flg"
  Relational Operator14/1 -> [VTQD_EngModeEnFlashFinished_flg]  "VTQD_EngModeEnFlashFinished_flg"
  Timer2/1 -> [VTQD_EngModeDisDetTime_s], Relational Operator12/1  "VTQD_EngModeDisDetTime_s"
  Constant26/1 -> Engineering Mode Enable Flasher/4(Cycle_cnt)
  SR_Latch10/1 -> [VTQD_FlasherDis_flg], Timer4/1, NOT10/1  "VTQD_FlasherDis_flg"
  Constant50/1 -> Switch15/1
  [VTQD_EngModeOnDelay_flg] -> Switch10/2
  [VTQD_InitLVchrgSvrMode_flg] -> Switch21/1
  Switch7/1 -> Switch15/3
  [VTQD_EngModeDisFlashFinished_flg] -> Delay12/1
  Add13/1 -> Product5/2
  Delay15/1 -> SR_Latch3/2
  Delay13/1 -> Switch11/3
  Constant45/1 -> Add14/1
  Add12/1 -> Product7/1  "VTQD_DisFlashCycleTime_s"
  Engineering Mode Enable Flasher/1(SigOut) -> Switch19/1
  Constant15/1 -> Timer1/4, Relational Operator10/2
  Constant34/1 -> Add13/1
  Constant43/1 -> Add12/2
  Product6/1 -> Add12/1
  Constant46/1 -> Switch20/3
  Switch11/1 -> Switch10/3
  AND11/1 -> Switch4/2, SR_Latch1/1
  Product5/1 -> Relational Operator14/2, Timer3/4
  Delay12/1 -> SR_Latch10/2
  Timer3/1 -> Relational Operator14/1
  Relational Operator10/1 -> [VTQD_EngModeEnDetEnd_flg]  "VTQD_EngModeEnDetEnd_flg"
  Constant44/1 -> Switch4/3
  [VTQD_EngModeDisFlashFinished_flg] -> OR1/1
  AND12/1 -> Switch8/2, SR_Latch2/1
  Constant51/1 -> Data Type Conversion8/1
  Constant49/1 -> Switch10/1
  Constant23/1 -> Data Type Conversion6/1
  Switch4/1 -> Add7/1
  Delay11/1 -> AND9/1
  Switch21/1 -> [VTQD_LVchrgSvrMode_flg], Delay14/1  "VTQD_LVchrgSvrMode_flg"
  Constant19/1 -> Engineering Mode Enable Flasher/2(ON_s)
  Constant25/1 -> Engineering Mode Enable Flasher/3(OFF_s)
  [VTQD_LVchrgSvrModeDelay_flg] -> AND12/2
  Timer4/1 -> Relational Operator15/1
  [VTQD_EngModeOffDelay_flg] -> Switch15/2
  Constant47/1 -> Add13/2
  [task_time_s] -> Timer3/3
  Product4/1 -> Add10/1
  SR_Latch2/1 -> Timer2/1, NOT8/1
  Constant48/1 -> Add14/2
  Constant52/1 -> Switch5/1
  [VTQD_EngModeEnFlashFinished_flg] -> Delay15/1
  [VTQD_FlasherDis_flg] -> Switch20/2
  Add14/1 -> Product7/2
  Constant176/1 -> Equal31/2
  [VACC_ASC2NLvReqFA_enum] -> Equal31/1
  Equal31/1 -> Detect Rise Positive2/1  "VTQD_EngModeOnSig_flg"
  [VTQD_EngModeOnRiseDet_flg] -> AND11/1
  Equal10/1 -> Detect Rise Positive1/1  "VTQD_EngModeOffSig_flg"
  [VACC_ASC2NLvReqFA_enum] -> Equal10/1
  Constant4/1 -> Equal10/2
  Detect Rise Positive1/1 -> [VTQD_EngModeOffRiseDet_flg]  "VTQD_EngModeOffRiseDet_flg"
  [VTQD_EngModeOffRiseDet_flg] -> AND12/1
  Switch19/1 -> [VTQD_AmberFlashOn_flg]  "VTQD_AmberFlashOn_flg"
  [task_time_s] -> "Big Mike Combo V2 "/1(task_time_s)
  [VACC_ASC2NLvReqFA_enum] -> "Big Mike Combo V2 "/2(VACC_ASC2NLvReqFA_enum)
  [VACC_ASC2NLvReqRA_enum] -> "Big Mike Combo V2 "/3(VACC_ASC2NLvReqRA_enum)
  [VACC_ASC2KneeReqRSide_flg] -> "Big Mike Combo V2 "/4(VACC_ASC2KneeReqRSide_flg)
  [VACC_ASC2KneeReqFA_flg] -> "Big Mike Combo V2 "/5(VACC_ASC2KneeReqFA_flg)
  [VACC_ASC2KneeReqRA_flg] -> "Big Mike Combo V2 "/6(VACC_ASC2KneeReqRA_flg)
  [VBCM_FDCBCMFDCloseSVCmd_flg] -> "Big Mike Combo V2 "/7(VBCM_FDCBCMFDCloseSVCmd_flg)
  [VBCM_FDCBCMFDOpenSVCmd_flg] -> "Big Mike Combo V2 "/8(VBCM_FDCBCMFDOpenSVCmd_flg)
  [VINP_TransReqGear_enum] -> "Big Mike Combo V2 "/9(VINP_TransReqGear_enum)
  [VINP_ParkBrakeSW_flg] -> "Big Mike Combo V2 "/10(VINP_ParkBrakeSW_flg)
  Bus Selector/29 -> [VINP_ParkBrakeSW_flg]  "<VINP_ParkBrakeSW_flg>"
  Bus Selector/30 -> [VINP_BrakePedalPos_pct]  "<VINP_BrakePedalPos_pct>"
  [VINP_BrakePedalPos_pct] -> "Big Mike Combo V2 "/11(VINP_BrakePedalPos_pct)
  [VDHP_ActAPSPosn_pct] -> "Big Mike Combo V2 "/12(VDHP_ActAPSPosn_pct)
  Bus Selector/31 -> [VDHP_ActAPSPosn_pct]  "<VDHP_ActAPSPosn_pct>"
  [VPMM_SysPowerMode_enum] -> "Big Mike Combo V2 "/13(VPMM_SysPowerMode_enum)
  [VTQD_GearActualPosn_enum] -> "Big Mike Combo V2 "/14(VTQD_GearActualPosn_enum)
  [VTQD_ActFRDoorOPSta_flg] -> "Big Mike Combo V2 "/15(VTQD_ActFRDoorOPSta_flg)
  "Big Mike Combo V2 "/1(VTQD_Function1Off_flg) -> [VTQD_Function1Off_flg]
  "Big Mike Combo V2 "/2(VTQD_Function2Off_flg) -> [VTQD_Function2Off_flg]
  "Big Mike Combo V2 "/3(VTQD_Function3Off_flg) -> [VTQD_Function3Off_flg]
  "Big Mike Combo V2 "/4(VTQD_Function4Off_flg) -> [VTQD_Function4Off_flg]
  "Big Mike Combo V2 "/5(VTQD_Function5Off_flg) -> [VTQD_Function5Off_flg]
  "Big Mike Combo V2 "/6(VTQD_ComboKeyEn_flg) -> [VTQD_ComboKeyEn_flg]
  "Big Mike Combo V2 "/7(VTQD_ComboKeyPreEn_flg) -> [VTQD_ComboKeyPreEn_flg]
  "Big Mike Combo V2 "/8(VTQD_FunctionOffSta_enum) -> [VTQD_FunctionOffSta_enum]
  [VDMM_DTCLostB2VST1_flg] -> OR2/1
  Bus Selector/32 -> [VDMM_DTCLostB2VST1_flg]  "<VDMM_DTCLostB2VST1_flg>"
  Bus Selector/33 -> [VDMM_DTCLostB2VST2_flg]  "<VDMM_DTCLostB2VST2_flg>"
  [VDMM_DTCLostB2VST2_flg] -> OR2/2
  Bus Selector/34 -> [VDMM_DTCLostB2VCurrentLimit_flg]  "<VDMM_DTCLostB2VCurrentLimit_flg>"
  [VDMM_DTCLostB2VCurrentLimit_flg] -> OR2/3
  OR2/1 -> [VTQD_LostComBCU_flg]  "VTQD_LostComBCU_flg"
  [VDMM_DTCLostTC1_flg] -> Data Type Conversion/1
  Data Type Conversion/1 -> [VTQD_LostComDMS_flg]  "VTQD_LostComDMS_flg"
  Bus Selector/35 -> [VDMM_DTCLostEMCEM1_flg]  "<VDMM_DTCLostEMCEM1_flg>"
  Bus Selector/36 -> [VDMM_DTCLostEBC1_flg]  "<VDMM_DTCLostEBC1_flg>"
  Bus Selector/37 -> [VDMM_DTCLostEBC2_flg]  "<VDMM_DTCLostEBC2_flg>"
  Bus Selector/38 -> [VDMM_DTCLostEBC5_flg]  "<VDMM_DTCLostEBC5_flg>"
  [VDMM_DTCLostEMCEM1_flg] -> OR3/1
  [VDMM_DTCLostEBC1_flg] -> OR3/2
  [VDMM_DTCLostEBC2_flg] -> OR3/3
  [VDMM_DTCLostEBC5_flg] -> OR3/4
  OR3/1 -> [VTQD_LostComEBS_flg]  "VTQD_LostComEBS_flg"
  OR4/1 -> [VTQD_LostComTempEBS_flg]  "VTQD_LostComTempEBS_flg"
  [VDMM_ActLostEBC5_flg] -> OR4/4
  [VDMM_ActLostEBC2_flg] -> OR4/3
  [VDMM_ActLostEBC1_flg] -> OR4/2
  [VDMM_ActLostEMCEM1_flg] -> OR4/1
  Bus Selector/39 -> [VDMM_ActLostEMCEM1_flg]  "<VDMM_ActLostEMCEM1_flg>"
  Bus Selector/40 -> [VDMM_ActLostEBC1_flg]  "<VDMM_ActLostEBC1_flg>"
  Bus Selector/41 -> [VDMM_ActLostEBC2_flg]  "<VDMM_ActLostEBC2_flg>"
  Bus Selector/42 -> [VDMM_ActLostEBC5_flg]  "<VDMM_ActLostEBC5_flg>"
  Bus Selector/43 -> [VDMM_ActLostMCUSta1_flg]  "<VDMM_ActLostMCUSta1_flg>"
  Bus Selector/44 -> [VDMM_ActLostMCUSta2_flg]  "<VDMM_ActLostMCUSta2_flg>"
  Bus Selector/45 -> [VDMM_ActLostMCUSta3_flg]  "<VDMM_ActLostMCUSta3_flg>"
  [VDMM_ActLostMCUSta1_flg] -> OR5/1
  OR5/1 -> [VTQD_LostComTempMCU_flg]  "VTQD_LostComTempMCU_flg"
  [VDMM_ActLostMCUSta3_flg] -> OR5/3
  [VDMM_ActLostMCUSta2_flg] -> OR5/2
  [VDMM_ActLostB2VST2_flg] -> OR6/2
  [VDMM_ActLostB2VCurrentLimit_flg] -> OR6/3
  OR6/1 -> [VTQD_LostComTempBCU_flg]  "VTQD_LostComTempBCU_flg"
  [VDMM_ActLostB2VST1_flg] -> OR6/1
  Bus Selector/46 -> [VDMM_ActLostB2VST1_flg]  "<VDMM_ActLostB2VST1_flg>"
  Bus Selector/47 -> [VDMM_ActLostB2VST2_flg]  "<VDMM_ActLostB2VST2_flg>"
  Bus Selector/48 -> [VDMM_ActLostB2VCurrentLimit_flg]  "<VDMM_ActLostB2VCurrentLimit_flg>"
  [VDMM_DTCBCURCIncorrect_flg] -> OR7/1
  OR7/1 -> [VTQD_SpdForceZero_flg]  "VTQD_SpdForceZero_flg"
  [VDMM_DTCPDURCIncorrect_flg] -> OR7/2
  Bus Selector/49 -> [VDMM_DTCBCURCIncorrect_flg]  "<VDMM_DTCBCURCIncorrect_flg>"
  Bus Selector/50 -> [VDMM_DTCPDURCIncorrect_flg]  "<VDMM_DTCPDURCIncorrect_flg>"
  [VDMM_DTCMCUCtrlMdNoFB_flg] -> OR7/3
  [VDMM_DTCMCUIGBNoFB_flg] -> OR7/4
  [VDMM_DTCMCUHVRlyNoFB_flg] -> OR7/5
  [VDMM_DTCBMSRlyNoFB_flg] -> OR7/6
  [VDMM_DTCBMSRlyNoFB_flg] -> OR8/6
  [VDMM_DTCMCUHVRlyNoFB_flg] -> OR8/5
  [VDMM_DTCMCUIGBNoFB_flg] -> OR8/4
  [VDMM_DTCMCUCtrlMdNoFB_flg] -> OR8/3
  [VDMM_DTCPDURCIncorrect_flg] -> OR8/2
  OR8/1 -> [VTQD_TrqForceZero_flg]  "VTQD_TrqForceZero_flg"
  [VDMM_DTCBCURCIncorrect_flg] -> OR8/1
  OR9/1 -> [VTQD_TrqLimit_flg]  "VTQD_TrqLimit_flg"
  [VDMM_DTCMotorTrqNoFB_flg] -> OR9/8
  [VDMM_DTCEHPSRlyNoFB_flg] -> OR9/7
  [VDMM_DTCEHPSInverNoFB_flg] -> OR9/6
  [VDMM_DTCEACRlyNoFB_flg] -> OR9/5
  [VDMM_DTCEACInverNoFB_flg] -> OR9/4
  [VDMM_DTCDCDCRlyNoFB_flg] -> OR9/3
  [VDMM_DTCDCDCInverNoFB_flg] -> OR9/2
  [VDMM_DTCACHVRlyNoFB_flg] -> OR9/1
  [VDMM_DTCACHVRlyNoFB_flg] -> OR10/1
  [VDMM_DTCDCDCInverNoFB_flg] -> OR10/2
  [VDMM_DTCDCDCRlyNoFB_flg] -> OR10/3
  [VDMM_DTCEACInverNoFB_flg] -> OR10/4
  [VDMM_DTCEACRlyNoFB_flg] -> OR10/5
  [VDMM_DTCEHPSInverNoFB_flg] -> OR10/6
  [VDMM_DTCEHPSRlyNoFB_flg] -> OR10/7
  [VDMM_DTCMotorSpdNoFB_flg] -> OR10/8
  OR10/1 -> [VTQD_SpdLimit_flg]  "VTQD_SpdLimit_flg"
  AND1/1 -> SR_Latch5/2
  Constant7/1 -> Relational Operator1/2
  SR_Latch5/1 -> [VTQD_DMSLossLimitGear_flg]  "VTQD_DMSLossLimitGear_flg"
  Relational Operator1/1 -> AND1/2
  [VTQD_VCUVehSpd_kph] -> Relational Operator1/1
  NOT5/1 -> AND1/1
  [VTQD_LostComDMS_flg] -> SR_Latch5/1, NOT5/1
  Constant56/1 -> Relational Operator18/2
  Constant13/1 -> Relational Operator17/2
  Constant61/1 -> Relational Operator19/2
  Constant59/1 -> LiuZgSwitch2/1
  [VTQD_GearActualPosn_enum] -> Relational Operator17/1
  Relational Operator2/1 -> Logical Operator2/1
  [VTQD_GearActualPosn_enum] -> Relational Operator16/1
  Constant14/1 -> Relational Operator2/2
  Constant9/1 -> Relational Operator20/2
  Relational Operator19/1 -> Logical Operator9/1
  Relational Operator17/1 -> Logical Operator4/1
  [VTQD_GearActualPosn_enum] -> Relational Operator2/1
  Constant60/1 -> LiuZgSwitch4/1
  LiuZgSwitch4/1 -> LiuZgSwitch2/3
  Relational Operator16/1 -> Logical Operator2/2
  [VTQD_DRTransfer_flg] -> NOT12/1
  NOT6/1 -> Logical Operator5/2
  Logical Operator2/1 -> Logical Operator3/1
  Logical Operator5/1 -> LiuZgSwitch4/2
  Logical Operator9/1 -> Logical Operator3/2
  LiuZgSwitch2/1 -> LiuZgSwitch1/3
  [VTQD_RrRampTq_Nm] -> Relational Operator19/1
  LiuZgSwitch1/1 -> [VTQD_TMRotateDirectionReq_enum], Unit Delay1/1  "VTQD_TMRotateDirectionReq_enum"
  Constant58/1 -> LiuZgSwitch1/1
  Relational Operator18/1 -> Logical Operator5/1
  [VTQD_RrRampTq_Nm] -> Relational Operator20/1
  [VTQD_GearActualPosn_enum] -> Relational Operator18/1
  Unit Delay1/1 -> LiuZgSwitch4/3
  Logical Operator4/1 -> LiuZgSwitch2/2
  Logical Operator3/1 -> LiuZgSwitch1/2
  [VTQD_DRTransfer_flg] -> NOT6/1
  Relational Operator20/1 -> Logical Operator9/2
  Constant8/1 -> Relational Operator16/2
  Detect Change3/1 -> Logical Operator10/2
  Relational Operator22/1 -> Detect Change3/1
  Relational Operator21/1 -> Detect Change2/1
  Constant62/1 -> Relational Operator22/2
  Constant63/1 -> Relational Operator21/2
  RegenLV_inc2/1 -> Relational Operator23/2
  Logical Operator10/1 -> SR_Latch6/1
  [VTQD_GearActualPosn_enum] -> Relational Operator22/1
  [VTQD_GearActualPosn_enum] -> Relational Operator21/1
  [VTQD_RrRampTq_Nm] -> Relational Operator23/1
  SR_Latch6/1 -> [VTQD_DRTransfer_flg]  "VTQD_DRTransfer_flg"
  Detect Change2/1 -> Logical Operator10/1
  Relational Operator23/1 -> SR_Latch6/2
  Relational Operator24/1 -> [VTQD_ActvDmpDisabReq_flg]  "VTQD_ActvDmpDisabReq_flg"
  [VTQD_TMRotateDirectionReq_enum] -> Relational Operator24/1
  Constant64/1 -> Relational Operator24/2
  NOT12/1 -> Logical Operator4/2
  OR14/1 -> [VTQD_ForceDischarge_flg]  "VTQD_ForceDischarge_flg"
  [VDMM_DTCMCUIGBNoFB_flg] -> OR14/2
  [VDMM_DTCMCUCtrlMdNoFB_flg] -> OR14/1
  Abs/1 -> Gain2/1, Gain1/1
  Gain2/1 -> [VTQD_TqTargetShaftRevSpd_rpm]  "VTQD_TqTargetShaftRevSpd_rpm"
  Gain1/1 -> [VTQD_TqTargetShaftDrivSpd_rpm]  "VTQD_TqTargetShaftDrivSpd_rpm"
  [VINP_MotorSpd_rpm] -> Abs/1
  Relational Operator26/1 -> Logical Operator7/2
  Logical Operator6/1 -> Switch1/2
  [VTQD_TqTargetShaftDrivSpd_rpm] -> Switch1/3
  [VTQD_TqTargetShaftRevSpd_rpm] -> Switch1/1
  [VTQD_GearActualPosn_enum] -> Relational Operator27/1
  [VTQD_TMRrotateDirection_enum] -> Relational Operator26/1
  Switch1/1 -> [VTQD_TqTargetShaftSpd_rpm]  "VTQD_TqTargetShaftSpd_rpm"
  [VTQD_TMRrotateDirection_enum] -> Relational Operator28/1
  Relational Operator28/1 -> Logical Operator11/2
  Logical Operator11/1 -> Logical Operator6/2
  Logical Operator7/1 -> Logical Operator6/1
  Constant65/1 -> Relational Operator25/2
  Relational Operator27/1 -> Logical Operator11/1
  Relational Operator25/1 -> Logical Operator7/1
  Constant69/1 -> Relational Operator28/2
  [VTQD_GearActualPosn_enum] -> Relational Operator25/1
  Constant67/1 -> Relational Operator27/2
  Constant66/1 -> Relational Operator26/2
  Switch6/1 -> Switch/3
  [VINP_MotorSpd_rpm] -> Equal13/1
  Switch/1 -> [VTQD_TMRrotateDirection_enum]  "VTQD_TMRrotateDirection_enum"
  Equal13/1 -> Switch6/2
  Constant75/1 -> Switch6/3
  Constant74/1 -> Switch6/1
  Constant71/1 -> Equal11/2
  Constant73/1 -> Equal13/2
  Equal11/1 -> Switch/2
  [VINP_MotorSpd_rpm] -> Equal11/1
  Constant72/1 -> Switch/1
  Constant70/1 -> Divide/2
  Constant76/1 -> Divide1/2
  Divide/1 -> [VTQD_PTAvailMotTq_Nm]  "VTQD_PTAvailMotTq_Nm"
  Divide1/1 -> [VTQD_PTAvailGenTq_Nm]  "VTQD_PTAvailGenTq_Nm"
  [VTQD_TMTqCapMot_Nm] -> Divide/1
  [VTQD_TMTqCapGen_Nm] -> Divide1/1
  Constant78/1 -> Switch22/1
  [VINP_ECPVCUDRM_enum] -> Equal14/1
  Equal14/1 -> Switch22/2
  [VTQD_AccelPedalDepressed_flg] -> NOT13/1
  Constant77/1 -> Equal14/2
  NOT13/1 -> Switch3/2
  [VINP_ECPVCUDRM_enum] -> Switch3/1
  Switch3/1 -> Delay4/1
  Switch22/1 -> [VTQD_ActDriveMode_enum]  "VTQD_ActDriveMode_enum"
  Delay4/1 -> Switch3/3, Switch22/3
  Bus Selector/51 -> [VINP_ECPVCUDRM_enum]  "<VINP_ECPVCUDRM_enum>"
  SR_Latch8/1 -> OR22/3
  Relational Operator33/1 -> AND14/2
  Relational Operator32/1 -> AND13/2
  Constant80/1 -> Relational Operator29/2
  SR_Latch7/1 -> OR22/2
  Constant83/1 -> Relational Operator33/2
  [VTQD_VCUVehSpd_kph] -> Relational Operator29/1
  AND14/1 -> SR_Latch8/2
  NOT17/1 -> AND14/1
  AND13/1 -> SR_Latch7/2
  Relational Operator31/1 -> AND4/2
  [VTQD_LostComEBS_flg] -> NOT15/1, SR_Latch/1
  SR_Latch/1 -> OR21/1, OR22/4
  NOT15/1 -> AND4/1
  Constant84/1 -> Relational Operator31/2
  AND/1 -> SR_Latch7/1
  [VTQD_VCUVehSpd_kph] -> Relational Operator31/1
  SR_Latch9/1 -> OR22/1
  OR22/1 -> [VTQD_ComLostZeroPwr_flg]  "VTQD_ComLostZeroPwr_flg"
  AND15/1 -> SR_Latch9/2
  [VTQD_LostComDMS_flg] -> NOT16/1
  [VTQD_LostComBCU_flg] -> NOT17/1, SR_Latch8/1
  NOT18/1 -> AND15/1
  NOT16/1 -> AND13/1
  [VTQD_VCUVehSpd_kph] -> Relational Operator30/1
  Constant85/1 -> Relational Operator32/2
  Relational Operator29/1 -> AND/2
  AND4/1 -> SR_Latch/2
  [VTQD_VCUVehSpd_kph] -> Relational Operator33/1
  [VTQD_VCUVehSpd_kph] -> Relational Operator32/1
  Relational Operator30/1 -> AND15/2
  [VTQD_LostComTempEBS_flg] -> OR21/2
  [VTQD_LostComTempMCU_flg] -> NOT18/1, SR_Latch9/1
  [VTQD_LostComDMS_flg] -> AND/1
  Constant86/1 -> Relational Operator30/2
  OR21/1 -> [VTQD_EBSLostZeroReg_flg]  "VTQD_EBSLostZeroReg_flg"
  AND16/1 -> [VTQD_ActCAN1BUSOFF_flg]  "VTQD_ActCAN1BUSOFF_flg"
  [VTQD_VCUVehSpd_kph] -> Relational Operator34/1
  [VDMM_CAN1BUSOFF_flg] -> AND16/1
  Constant89/1 -> Relational Operator34/2
  Relational Operator34/1 -> AND16/2
  Bus Selector/52 -> [VDMM_CAN1BUSOFF_flg]  "<VDMM_CAN1BUSOFF_flg>"
  [VTQD_EBSLostZeroReg_flg] -> Switch24/2
  Constant90/1 -> Switch23/1
  [VINP_EM1OvrCtrlMBrk_enum] -> Equal/1
  Equal16/1 -> [VTQD_EM1LimitCtrlDriv_flg]  "VTQD_EM1LimitCtrlDriv_flg"
  Constant97/1 -> Equal16/2
  [VINP_EM1OvrCtrlMDriv_enum] -> Equal18/1
  Constant94/1 -> Equal17/2
  [VINP_EM1OvrCtrlMBrk_enum] -> Equal17/1
  Constant92/1 -> Equal/2
  Equal18/1 -> [VTQD_EM1TorqueCtrlDriv_flg]  "VTQD_EM1TorqueCtrlDriv_flg"
  Constant96/1 -> Equal18/2
  Switch24/1 -> [VTQD_EM1LimitCtrlBrk_flg]  "VTQD_EM1LimitCtrlBrk_flg"
  Equal17/1 -> Switch24/3
  [VINP_EM1OvrCtrlMDriv_enum] -> Equal16/1
  Constant98/1 -> Switch24/1
  [VTQD_EBSLostZeroReg_flg] -> Switch23/2
  Equal/1 -> Switch23/3
  Switch23/1 -> [VTQD_EM1TorqueCtrlBrk_flg]  "VTQD_EM1TorqueCtrlBrk_flg"
  Bus Selector/53 -> [VINP_EM1OvrCtrlMDriv_enum]  "<VINP_EM1OvrCtrlMDriv_enum>"
  Bus Selector/54 -> [VINP_EM1OvrCtrlMBrk_enum]  "<VINP_EM1OvrCtrlMBrk_enum>"
  [VTQD_TorqLimDoorOpn_flg] -> OR23/3
  [VTQD_ComLostZeroPwr_flg] -> OR23/4
  [VTQD_VCUMCUCtrlMd_enum] -> Relational Operator36/1
  Relational Operator36/1 -> OR23/2
  [VTQD_TrqForceZero_flg] -> OR23/5
  OR23/1 -> [VTQD_TrqCMDForveZero_flg]  "VTQD_TrqCMDForveZero_flg"
  Constant100/1 -> Relational Operator36/2
  Relational Operator35/1 -> OR23/1
  Constant99/1 -> Relational Operator35/2
  [VTQD_GearActualPosn_enum] -> Relational Operator35/1
  LiuZgSwitch7/1 -> [VTQD_TqSource_enum]  "VTQD_TqSource_enum"
  [VTQD_ComLostZeroPwr_flg] -> OR18/2
  OR15/1 -> OR20/2
  LiuZgSwitch6/1 -> LiuZgSwitch7/3
  [VTQD_EBSLostZeroReg_flg] -> OR18/3
  [VTQD_EM1TorqueCtrlDriv_flg] -> OR15/2
  NOT14/1 -> OR20/1
  Constant81/1 -> LiuZgSwitch7/1
  OR20/1 -> LiuZgSwitch7/2
  [VTQD_ComLostZeroPwr_flg] -> OR18/1
  [VTQD_EM1TorqueCtrlBrk_flg] -> OR15/1
  Constant79/1 -> LiuZgSwitch6/3
  Constant82/1 -> LiuZgSwitch6/1
  [VDMM_EBSRCIncorrect_flg] -> NOT14/1
  OR18/1 -> LiuZgSwitch6/2
  Bus Selector/55 -> [VDMM_EBSRCIncorrect_flg]  "<VDMM_EBSRCIncorrect_flg>"
  Constant102/1 -> AND17/1
  LiuZgSwitch8/1 -> [VTQD_TMSpd_rpm]  "VTQD_TMSpd_rpm"
  Equal15/1 -> AND17/2
  [VTQD_GearActualPosn_enum] -> Equal15/1
  Constant101/1 -> Equal15/2
  Gain3/1 -> LiuZgSwitch8/1
  AND17/1 -> LiuZgSwitch8/2
  [VINP_MotorSpd_rpm] -> Gain3/1
  [VINP_MotorSpd_rpm] -> LiuZgSwitch8/3
  [VTQD_TrqForceZero_flg] -> Bus Creator/42
  [VTQD_Function4Off_flg] -> Bus Creator/30
  [VTQD_DMSLossLimitGear_flg] -> Bus Creator/45
  [VTQD_EBSLostZeroReg_flg] -> Bus Creator/55
  [VTQD_NeutralPositionOn_flg] -> Bus Creator/5
  [VTQD_LVchrgSvrMode_flg] -> Bus Creator/22
  [VTQD_EVDriveReady_flg] -> Bus Creator/7
  [VTQD_EngModeDisDetTime_s] -> Bus Creator/23
  [VTQD_LostComDMS_flg] -> Bus Creator/36
  [VTQD_DRTransfer_flg] -> Bus Creator/46
  [VTQD_LostComTempMCU_flg] -> Bus Creator/39
  [VTQD_ActMDDoorOPSta_flg] -> Bus Creator/12
  [VTQD_Function2Off_flg] -> Bus Creator/28
  [VTQD_ComboKeyEn_flg] -> Bus Creator/32
  [VTQD_DrivePositionOn_flg] -> Bus Creator/4
  [VTQD_EM1LimitCtrlBrk_flg] -> Bus Creator/57
  [VTQD_AmberFlashOn_flg] -> Bus Creator/25
  [VTQD_AmberFlashOff_flg] -> Bus Creator/26
  [VTQD_EM1LimitCtrlDriv_flg] -> Bus Creator/60
  [VTQD_PTAvailGenTq_Nm] -> Bus Creator/52
  [VTQD_ActFRDoorOPSta_flg] -> Bus Creator/11
  Bus Creator/1 -> BSignalConvert_outputs/1  "BSignalConvert_outputs"
  [VTQD_LostComTempEBS_flg] -> Bus Creator/38
  [VTQD_Function5Off_flg] -> Bus Creator/31
  [VTQD_EngModeEnDetTime_s] -> Bus Creator/20
  [VTQD_DoorOpen_flg] -> Bus Creator/3
  [VTQD_FunctionOffSta_enum] -> Bus Creator/34
  [VTQD_EM1TorqueCtrlDriv_flg] -> Bus Creator/59
  [VTQD_EM1ReqTorqLimBrk_Nm] -> Bus Creator/10
  [VTQD_ForceDischarge_flg] -> Bus Creator/49
  [VTQD_TqTargetShaftSpd_rpm] -> Bus Creator/50
  [VTQD_ActvDmpDisabReq_flg] -> Bus Creator/48
  [VTQD_ActTDDoorOPSta_flg] -> Bus Creator/13
  [VTQD_SpdLimSta_flg] -> Bus Creator/19
  [VTQD_EngModeEnDetEnd_flg] -> Bus Creator/21
  [VTQD_EVCU1VehActDrvDir_enum] -> Bus Creator/17
  [VTQD_PTAvailMotTq_Nm] -> Bus Creator/51
  [VTQD_LostComBCU_flg] -> Bus Creator/35
  [VTQD_SpdLimit_flg] -> Bus Creator/44
  [VTQD_TMRotateDirectionReq_enum] -> Bus Creator/47
  [VTQD_Function1Off_flg] -> Bus Creator/27
  [VTQD_VCU4PweLmtInd_flg] -> Bus Creator/14
  [VTQD_EngModeDisDetEnd_flg] -> Bus Creator/24
  [VTQD_IGNActive_flg] -> Bus Creator/8
  [VTQD_TqSource_enum] -> Bus Creator/62
  [VTQD_GearFlashIndDis_flg] -> Bus Creator/15
  [VTQD_TrqCMDForveZero_flg] -> Bus Creator/61
  [VTQD_ActDriveMode_enum] -> Bus Creator/53
  [VTQD_ComLostZeroPwr_flg] -> Bus Creator/54
  [VTQD_SpdForceZero_flg] -> Bus Creator/41
  [VTQD_ActCAN1BUSOFF_flg] -> Bus Creator/56
  [VTQD_AccelPedalDepressed_flg] -> Bus Creator/1
  [VTQD_Function3Off_flg] -> Bus Creator/29
  [VTQD_ReversePositionOn_flg] -> Bus Creator/6
  [VTQD_GearFlashInd_flg] -> Bus Creator/16
  [VTQD_EM1ReqTorqLimDriv_Nm] -> Bus Creator/9
  [VTQD_ComboKeyPreEn_flg] -> Bus Creator/33
  [VTQD_LostComEBS_flg] -> Bus Creator/37
  [VTQD_LostComTempBCU_flg] -> Bus Creator/40
  [VTQD_BrkSWOn_flg] -> Bus Creator/2
  [VTQD_VCUMCUDemHiPosVal_rpm] -> Bus Creator/18
  [VTQD_TMSpd_rpm] -> Bus Creator/63
  [VTQD_TrqLimit_flg] -> Bus Creator/43
  [VTQD_EM1TorqueCtrlBrk_flg] -> Bus Creator/58
  Bus Selector/56 -> [VINP_FRHalbrakeReq_enum]  "<VINP_FRHalbrakeReq_enum>"
  Bus Selector/57 -> [VINP_MDHalbrakeReq_enum]  "<VINP_MDHalbrakeReq_enum>"
  Bus Selector/58 -> [VINP_TDHalbrakeReq_enum]  "<VINP_TDHalbrakeReq_enum>"
  Bus Selector/59 -> [VBCM_FDCBCMFDoorSta_flg]  "<VBCM_FDCBCMFDoorSta_flg>"
  Bus Selector/60 -> [VBCM_FDCBCMMDoorSta_flg]  "<VBCM_FDCBCMMDoorSta_flg>"
  Bus Selector/61 -> [VBCM_FDCBCMRDoorSta_flg]  "<VBCM_FDCBCMRDoorSta_flg>"
  Bus Selector/62 -> [VACC_ASC2NLvReqFA_enum]  "<VACC_ASC2NLvReqFA_enum>"
  Bus Selector/63 -> [VACC_ASC2NLvReqRA_enum]  "<VACC_ASC2NLvReqRA_enum>"
  Bus Selector/64 -> [VACC_ASC2KneeReqRSide_flg]  "<VACC_ASC2KneeReqRSide_flg>"
  Bus Selector/65 -> [VACC_ASC2KneeReqFA_flg]  "<VACC_ASC2KneeReqFA_flg>"
  Bus Selector/66 -> [VACC_ASC2KneeReqRA_flg]  "<VACC_ASC2KneeReqRA_flg>"
  Bus Selector/67 -> [VBCM_FDCBCMFDCloseSVCmd_flg]  "<VBCM_FDCBCMFDCloseSVCmd_flg>"
  Bus Selector/68 -> [VBCM_FDCBCMFDOpenSVCmd_flg]  "<VBCM_FDCBCMFDOpenSVCmd_flg>"
  BDCQ_Function_outputs/1 -> Bus Selector1/1
  Bus Selector1/1 -> [VTQD_GearActualPosn_enum]  "<VTQD_GearActualPosn_enum>"
  Bus Selector1/2 -> [VTQD_ParkingProtectWarning_flg]  "<VTQD_ParkingProtectWarning_flg>"
  Bus Selector1/3 -> [VTQD_TorqLimDoorOpn_flg]  "<VTQD_TorqLimDoorOpn_flg>"
  Bus Selector1/4 -> [VTQD_VCUMCUCtrlMd_enum]  "<VTQD_VCUMCUCtrlMdTQD_enum>"
  Max/1 -> Engineering Mode Enable Flasher/1(Task_Time_s)
  [task_time_s] -> Max/1
  Constant103/1 -> Max/2
  Constant111/1 -> Max1/2
  Max1/1 -> Engineering Mode Disable Flasher/1(Task_Time_s)
  [task_time_s] -> Max1/1
  Delay5/1 -> Equal7/1
  Delay6/1 -> Equal3/1
  [VTQD_GearActualPosn_enum] -> Delay6/1
  Constant104/1 -> Equal3/2
  [VTQD_GearActualPosn_enum] -> Delay5/1
  Constant105/1 -> Equal7/2
  BDCQ_main_outputs/1 -> Bus Selector2/1
  Bus Selector2/1 -> [VTQD_RrRampTq_Nm]  "<VTQD_RrRampTq_Nm>"
  Constant114/1 -> Max2/1
  Constant117/1 -> Max2/2
  Max2/1 -> Divide2/2
  [VINP_MotorSpd_rpm] -> Divide2/1
  Divide2/1 -> Product8/1
  Constant122/1 -> Product8/2
  Constant118/1 -> Product8/3
  Constant119/1 -> Product8/4
  Constant120/1 -> Product8/5
  Constant123/1 -> Max3/1
  Constant124/1 -> Max3/2
  Max3/1 -> Divide3/2
  Product8/1 -> Divide3/1
  Data Type Conversion1/1 -> Abs1/1
  Divide3/1 -> Data Type Conversion1/1
  Abs1/1 -> [VTQD_VCUTMVehSpd_kph]  "VTQD_VCUTMVehSpd_kph"
  AND18/1 -> Switch28/2
  [VTQD_VCUTMVehSpd_kph] -> Switch28/3
  Relational Operator37/1 -> AND18/3
  Bus Selector/69 -> [VINP_FASpeed_kph]  "<VINP_FASpeed_kph>"
  [VINP_FASpeed_kph] -> Relational Operator37/1
  Constant125/1 -> Relational Operator37/2
  [VINP_FASpeed_kph] -> Relational Operator38/1
  Constant126/1 -> Relational Operator38/2
  Bus Selector/70 -> [VINP_CANMsgValidEBC2_flg]  "<VINP_CANMsgValidEBC2_flg>"
  Relational Operator38/1 -> AND18/1
  [VINP_CANMsgValidEBC2_flg] -> AND18/2
  [VINP_FASpeed_kph] -> Switch28/1
  Switch28/1 -> [VTQD_VCUVehSpd_kph]  "VTQD_VCUVehSpd_kph"
  [VTQD_VCUTMVehSpd_kph] -> Bus Creator/64
  [VTQD_VCUVehSpd_kph] -> Bus Creator/65
  Bus Selector1/5 -> [VTQD_TMTqCapMot_Nm]  "<VTQD_TMTqCapMot_Nm>"
  Bus Selector1/6 -> [VTQD_TMTqCapGen_Nm]  "<VTQD_TMTqCapGen_Nm>"
  Data Type Conversion6/1 -> Relational Operator13/2
  Data Type Conversion4/1 -> Relational Operator13/1
  Data Type Conversion7/1 -> Relational Operator11/1
  Data Type Conversion8/1 -> Relational Operator11/2
